simulink model "nonlinearstm_c"  (R2018b)
settings: configuration reference "Physics" (kept outside this file)
model workspace (MAT data in the model file):
  x0_positionstates = Simulink.Parameter
  x0_positionstates.Value = [0 0 0]
  x0_positionstates.DataType = 'auto'
  x0_positionstates.Dimensions = [1 3]
undefined symbols (not defined in the file): INIT__initialvalues__omega0_Wheels_radps__1, INIT__initialvalues__omega0_Wheels_radps__2, INIT__initialvalues__omega0_Wheels_radps__3, INIT__initialvalues__omega0_Wheels_radps__4, INIT__initialvalues__Vehicle_InitialVelocity_mps__1, INIT__initialvalues__Vehicle_InitialVelocity_mps__2, INIT__initialvalues__Vehicle_InitialYawRate_radps, x0_stm_vehiclestates
settings Model: DataDictionary=vehicleparameters_vehdynsim.sldd  OrderedModelArguments=off  Creator=wischnewski  LastModifiedBy=jens

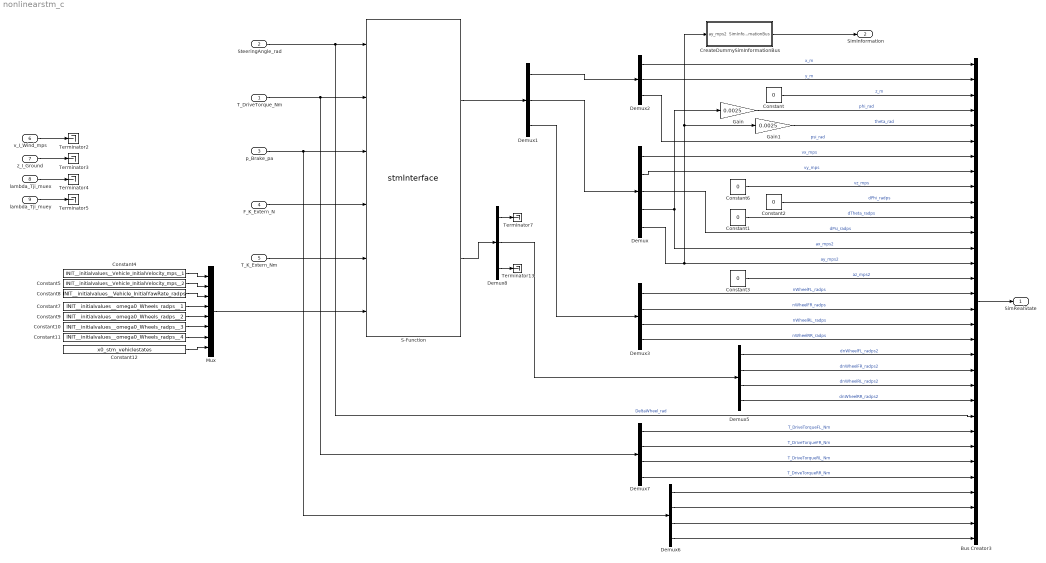
== system nonlinearstm_c ==
  T_DriveTorque_Nm : Inport
  SteeringAngle_rad : Inport  Port=2
  p_Brake_pa : Inport  Port=3
  F_K_Extern_N : Inport  Port=4  PortDimensions=3
  T_K_Extern_Nm : Inport  Port=5  PortDimensions=3
  v_I_Wind_mps : Inport  Port=6  PortDimensions=3
  z_I_Ground : Inport  Port=7  PortDimensions=4
  lambda_Tji_muex : Inport  Port=8  PortDimensions=4
  lambda_Tji_muey : Inport  Port=9  PortDimensions=4
  Bus Creator3 : BusCreator  Inputs=32  OutDataTypeStr=Bus: SimRealState
  Constant{,1..3,6} (5 alike) : Constant  Value=0
  Constant10 : Constant  Value=INIT__initialvalues__omega0_Wheels_radps__3
  Constant11 : Constant  Value=INIT__initialvalues__omega0_Wheels_radps__4
  Constant12 : Constant  Value=x0_stm_vehiclestates
  Constant4 : Constant  Value=INIT__initialvalues__Vehicle_InitialVelocity_mps__1
  Constant5 : Constant  Value=INIT__initialvalues__Vehicle_InitialVelocity_mps__2
  Constant7 : Constant  Value=INIT__initialvalues__omega0_Wheels_radps__1
  Constant8 : Constant  Value=INIT__initialvalues__Vehicle_InitialYawRate_radps
  Constant9 : Constant  Value=INIT__initialvalues__omega0_Wheels_radps__2
  CreateDummySimInformationBus : Subsystem
  Demux : Demux  Outputs=[1 1 1 1 1]
  Demux1 : Demux  Outputs=[3 5 4]
  Demux2 : Demux  Outputs=3
  Demux{3,5..7} (4 alike) : Demux
  Demux8 : Demux  Outputs=[6 4 8]
  Gain : Gain  Gain=0.0025
  Gain1 : Gain  Gain=0.0025
  Mux : Mux  Inputs=8
  S-Function : S-Function  FunctionName=stmInterface  SFunctionDeploymentMode=off  EnableBusSupport=off
  Terminator{2..5,7,13} (6 alike) : Terminator
  SimRealState : Outport  OutDataTypeStr=Bus: SimRealState
  SimInformation : Outport  Port=2  OutDataTypeStr=Bus: SimInformation
  wires:
  Demux/1 -> Bus Creator3/7  "vx_mps"
  Demux/2 -> Bus Creator3/8  "vy_mps"
  Demux2/3 -> Bus Creator3/6  "psi_rad"
  Demux/3 -> Bus Creator3/12  "dPsi_radps"
  Demux/4 -> Gain/1, Bus Creator3/13  "ax_mps2"
  Demux/5 -> Bus Creator3/14, CreateDummySimInformationBus/1(ay_mps2), Gain1/1  "ay_mps2"
  Demux2/1 -> Bus Creator3/1  "x_m"
  Demux2/2 -> Bus Creator3/2  "y_m"
  SteeringAngle_rad/1 -> Bus Creator3/24, S-Function/1  "DeltaWheel_rad"
  Bus Creator3/1 -> SimRealState/1
  Demux3/1 -> Bus Creator3/16  "nWheelFL_radps"
  Demux3/2 -> Bus Creator3/17  "nWheelFR_radps"
  Demux3/4 -> Bus Creator3/19  "nWheelRR_radps"
  Demux3/3 -> Bus Creator3/18  "nWheelRL_radps"
  Constant1/1 -> Bus Creator3/11  "dTheta_radps"
  Constant2/1 -> Bus Creator3/10  "dPhi_radps"
  Constant3/1 -> Bus Creator3/15  "az_mps2"
  Constant/1 -> Bus Creator3/3  "z_m"
  Gain1/1 -> Bus Creator3/5  "theta_rad"
  Gain/1 -> Bus Creator3/4  "phi_rad"
  Constant6/1 -> Bus Creator3/9  "vz_mps"
  T_DriveTorque_Nm/1 -> Demux7/1, S-Function/2
  p_Brake_pa/1 -> Demux6/1, S-Function/3
  v_I_Wind_mps/1 -> Terminator2/1
  z_I_Ground/1 -> Terminator3/1
  lambda_Tji_muex/1 -> Terminator4/1
  lambda_Tji_muey/1 -> Terminator5/1
  Demux5/2 -> Bus Creator3/21  "dnWheelFR_radps2"
  Demux5/3 -> Bus Creator3/22  "dnWheelRL_radps2"
  Demux5/4 -> Bus Creator3/23  "dnWheelRR_radps2"
  Demux5/1 -> Bus Creator3/20  "dnWheelFL_radps2"
  CreateDummySimInformationBus/1(SimInformationBus) -> SimInformation/1
  Demux7/1 -> Bus Creator3/25  "T_DriveTorqueFL_Nm"
  Demux7/2 -> Bus Creator3/26  "T_DriveTorqueFR_Nm"
  Demux7/3 -> Bus Creator3/27  "T_DriveTorqueRL_Nm"
  Demux7/4 -> Bus Creator3/28  "T_DriveTorqueRR_Nm"
  Demux6/1 -> Bus Creator3/29
  Demux6/2 -> Bus Creator3/30
  Demux6/3 -> Bus Creator3/31
  Demux6/4 -> Bus Creator3/32
  Mux/1 -> S-Function/6
  Constant5/1 -> Mux/2
  Constant4/1 -> Mux/1
  Constant8/1 -> Mux/3
  Constant7/1 -> Mux/4
  Constant9/1 -> Mux/5
  Constant10/1 -> Mux/6
  Constant11/1 -> Mux/7
  Constant12/1 -> Mux/8
  F_K_Extern_N/1 -> S-Function/4
  T_K_Extern_Nm/1 -> S-Function/5
  S-Function/1 -> Demux1/1
  Demux1/1 -> Demux2/1
  Demux1/2 -> Demux/1
  Demux1/3 -> Demux3/1
  S-Function/2 -> Demux8/1
  Demux8/1 -> Terminator7/1
  Demux8/3 -> Terminator13/1
  Demux8/2 -> Demux5/1

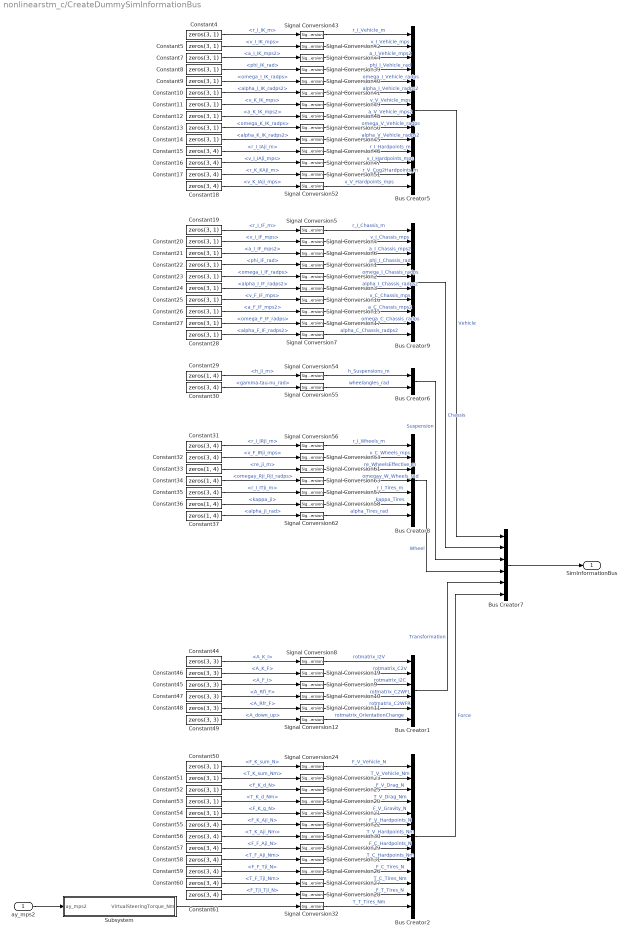
== system nonlinearstm_c/CreateDummySimInformationBus ==
  ay_mps2 : Inport
  Bus Creator1 : BusCreator  Inputs=6  OutDataTypeStr=Bus: Transformation
      settings: InheritFromInputs=off
  Bus Creator2 : BusCreator  Inputs=13  OutDataTypeStr=Bus: Force
      settings: InheritFromInputs=off
  Bus Creator5 : BusCreator  Inputs=14  OutDataTypeStr=Bus: Vehicle
      settings: InheritFromInputs=off
  Bus Creator6 : BusCreator  Inputs=2  OutDataTypeStr=Bus: Suspension
      settings: InheritFromInputs=off
  Bus Creator7 : BusCreator  Inputs=6  OutDataTypeStr=Bus: SimInformation
      settings: InheritFromInputs=off
  Bus Creator8 : BusCreator  Inputs=7  OutDataTypeStr=Bus: Wheel
      settings: InheritFromInputs=off
  Bus Creator9 : BusCreator  Inputs=10  OutDataTypeStr=Bus: Chassis
      settings: InheritFromInputs=off
  Constant{4..5,7..14,19..28,50..54} (25 alike) : Constant  Value=zeros(3, 1)
  Constant{15..18,30..32,35,55..61} (15 alike) : Constant  Value=zeros(3, 4)
  Constant{29,33..34,36..37} (5 alike) : Constant  Value=zeros(1, 4)
  Constant{44..49} (6 alike) : Constant  Value=zeros(3, 3)
  Signal Conversion{1..12,15..17,19..32,39..58,61..63} (52 alike) : SignalConversion  OverrideOpt=off
  Subsystem : Subsystem
  SimInformationBus : Outport
  wires:
  Signal Conversion46/1 -> Bus Creator5/11  "r_I_Hardpoints_m"
  Signal Conversion26/1 -> Bus Creator2/10  "F_C_Tires_N"
  Signal Conversion45/1 -> Bus Creator5/10  "alpha_V_Vehicle_radps2"
  Constant33/1 -> Signal Conversion61/1  "<re_ji_m>"
  Signal Conversion15/1 -> Bus Creator9/8  "a_C_Chassis_mps2"
  Signal Conversion58/1 -> Bus Creator8/6  "kappa_Tires"
  Constant60/1 -> Signal Conversion27/1  "<T_F_Tji_Nm>"
  Signal Conversion5/1 -> Bus Creator9/1  "r_I_Chassis_m"
  Signal Conversion17/1 -> Bus Creator9/9  "omega_C_Chassis_radps"
  Signal Conversion8/1 -> Bus Creator1/1  "rotmatrix_I2V"
  Constant13/1 -> Signal Conversion50/1  "<omega_K_IK_radps>"
  Constant24/1 -> Signal Conversion3/1  "<alpha_I_IF_radps2>"
  Signal Conversion16/1 -> Bus Creator9/7  "v_C_Chassis_mps"
  Signal Conversion23/1 -> Bus Creator2/2  "T_V_Vehicle_Nm"
  Signal Conversion3/1 -> Bus Creator9/6  "alpha_I_Chassis_radps2"
  Bus Creator5/1 -> Bus Creator7/1  "Vehicle"
  Signal Conversion32/1 -> Bus Creator2/13  "T_T_Tires_Nm"
  Signal Conversion39/1 -> Bus Creator5/4  "phi_I_Vehicle_rad"
  Signal Conversion29/1 -> Bus Creator2/8  "F_C_Hardpoints_N"
  Constant25/1 -> Signal Conversion16/1  "<v_F_IF_mps>"
  Signal Conversion43/1 -> Bus Creator5/1  "r_I_Vehicle_m"
  Constant47/1 -> Signal Conversion10/1  "<A_Rfl_F>"
  Constant9/1 -> Signal Conversion40/1  "<omega_I_IK_radps>"
  Constant26/1 -> Signal Conversion15/1  "<a_F_IF_mps2>"
  Constant27/1 -> Signal Conversion17/1  "<omega_F_IF_radps>"
  Signal Conversion10/1 -> Bus Creator1/4  "rotmatrix_C2WFL"
  Signal Conversion19/1 -> Bus Creator1/2  "rotmatrix_C2V"
  Constant7/1 -> Signal Conversion44/1  "<a_I_IK_mps2>"
  Bus Creator8/1 -> Bus Creator7/4  "Wheel"
  Signal Conversion9/1 -> Bus Creator1/3  "rotmatrix_I2C"
  Signal Conversion31/1 -> Bus Creator2/9  "T_C_Hardpoints_Nm"
  Signal Conversion62/1 -> Bus Creator8/7  "alpha_Tires_rad"
  Signal Conversion30/1 -> Bus Creator2/7  "T_V_Hardpoints_Nm"
  Signal Conversion48/1 -> Bus Creator5/8  "a_V_Vehicle_mps2"
  Signal Conversion54/1 -> Bus Creator6/1  "h_Suspensions_m"
  Signal Conversion56/1 -> Bus Creator8/1  "r_I_Wheels_m"
  Signal Conversion7/1 -> Bus Creator9/10  "alpha_C_Chassis_radps2"
  Signal Conversion12/1 -> Bus Creator1/6  "rotmatrix_OrientationChange"
  Signal Conversion21/1 -> Bus Creator2/5  "F_V_Gravity_N"
  Signal Conversion53/1 -> Bus Creator8/2  "v_C_Wheels_mps"
  Signal Conversion22/1 -> Bus Creator2/6  "F_V_Hardpoints_N"
  Signal Conversion27/1 -> Bus Creator2/11  "T_C_Tires_Nm"
  Signal Conversion51/1 -> Bus Creator5/13  "r_V_Cog2Hardpoints_m"
  Constant28/1 -> Signal Conversion7/1  "<alpha_F_IF_radps2>"
  Signal Conversion55/1 -> Bus Creator6/2  "wheelangles_rad"
  Signal Conversion57/1 -> Bus Creator8/5  "r_I_Tires_m"
  Signal Conversion4/1 -> Bus Creator9/2  "v_I_Chassis_mps"
  Bus Creator2/1 -> Bus Creator7/6  "Force"
  Signal Conversion20/1 -> Bus Creator2/4  "T_V_Drag_Nm"
  Signal Conversion40/1 -> Bus Creator5/5  "omega_I_Vehicle_radps"
  Bus Creator1/1 -> Bus Creator7/5  "Transformation"
  Signal Conversion41/1 -> Bus Creator5/6  "alpha_I_Vehicle_radps2"
  Bus Creator9/1 -> Bus Creator7/2  "Chassis"
  Signal Conversion6/1 -> Bus Creator9/3  "a_I_Chassis_mps2"
  Bus Creator6/1 -> Bus Creator7/3  "Suspension"
  Signal Conversion61/1 -> Bus Creator8/3  "re_WheelsEffective_m"
  Signal Conversion44/1 -> Bus Creator5/3  "a_I_Vehicle_mps2"
  Signal Conversion42/1 -> Bus Creator5/2  "v_I_Vehicle_mps"
  Signal Conversion63/1 -> Bus Creator8/4  "omegay_W_Wheels_rad"
  Constant31/1 -> Signal Conversion56/1  "<r_I_IRji_m>"
  Signal Conversion49/1 -> Bus Creator5/7  "v_V_Vehicle_mps"
  Signal Conversion28/1 -> Bus Creator2/12  "F_T_Tires_N"
  Signal Conversion11/1 -> Bus Creator1/5  "rotmatrix_C2WFR"
  Signal Conversion50/1 -> Bus Creator5/9  "omega_V_Vehicle_radps"
  Signal Conversion24/1 -> Bus Creator2/1  "F_V_Vehicle_N"
  Constant19/1 -> Signal Conversion5/1  "<r_I_IF_m>"
  Constant22/1 -> Signal Conversion1/1  "<phi_IF_rad>"
  Constant11/1 -> Signal Conversion49/1  "<v_K_IK_mps>"
  Constant58/1 -> Signal Conversion31/1  "<T_F_Aji_Nm>"
  Constant20/1 -> Signal Conversion4/1  "<v_I_IF_mps>"
  Constant44/1 -> Signal Conversion8/1  "<A_K_I>"
  Constant36/1 -> Signal Conversion58/1  "<kappa_ji>"
  Constant32/1 -> Signal Conversion53/1  "<v_F_IRji_mps>"
  Constant8/1 -> Signal Conversion39/1  "<phi_IK_rad>"
  Signal Conversion2/1 -> Bus Creator9/5  "omega_I_Chassis_radps"
  Constant5/1 -> Signal Conversion42/1  "<v_I_IK_mps>"
  Constant10/1 -> Signal Conversion41/1  "<alpha_I_IK_radps2>"
  Constant4/1 -> Signal Conversion43/1  "<r_I_IK_m>"
  Constant29/1 -> Signal Conversion54/1  "<h_ji_m>"
  Subsystem/1(VirtualSteeringTorque_Nm) -> Signal Conversion32/1
  Constant35/1 -> Signal Conversion57/1  "<r_I_ITji_m>"
  Signal Conversion47/1 -> Bus Creator5/12  "v_I_Hardpoints_mps"
  Constant57/1 -> Signal Conversion29/1  "<F_F_Aji_N>"
  Constant48/1 -> Signal Conversion11/1  "<A_Rfr_F>"
  Constant50/1 -> Signal Conversion24/1  "<F_K_sum_N>"
  Constant53/1 -> Signal Conversion20/1  "<T_K_d_Nm>"
  Constant49/1 -> Signal Conversion12/1  "<A_down_up>"
  Constant51/1 -> Signal Conversion23/1  "<T_K_sum_Nm>"
  Constant12/1 -> Signal Conversion48/1  "<a_K_IK_mps2>"
  Constant15/1 -> Signal Conversion46/1  "<r_I_IAji_m>"
  Constant54/1 -> Signal Conversion21/1  "<F_K_g_N>"
  Constant17/1 -> Signal Conversion51/1  "<r_K_KAji_m>"
  Constant55/1 -> Signal Conversion22/1  "<F_K_Aji_N>"
  Constant21/1 -> Signal Conversion6/1  "<a_I_IF_mps2>"
  Constant52/1 -> Signal Conversion25/1  "<F_K_d_N>"
  Constant30/1 -> Signal Conversion55/1  "<gamma-tau-nu_rad>"
  Constant14/1 -> Signal Conversion45/1  "<alpha_K_IK_radps2>"
  Constant18/1 -> Signal Conversion52/1  "<v_K_IAji_mps>"
  Constant59/1 -> Signal Conversion26/1  "<F_F_Tji_N>"
  Constant61/1 -> Signal Conversion28/1  "<F_Tji_Tji_N>"
  Constant56/1 -> Signal Conversion30/1  "<T_K_Aji_Nm>"
  Constant37/1 -> Signal Conversion62/1  "<alpha_ji_rad>"
  Constant34/1 -> Signal Conversion63/1  "<omegay_Rji_Rji_radps>"
  Constant45/1 -> Signal Conversion9/1  "<A_F_I>"
  Signal Conversion1/1 -> Bus Creator9/4  "phi_I_Chassis_rad"
  Signal Conversion52/1 -> Bus Creator5/14  "v_V_Hardpoints_mps"
  Constant46/1 -> Signal Conversion19/1  "<A_K_F>"
  Constant23/1 -> Signal Conversion2/1  "<omega_I_IF_radps>"
  Constant16/1 -> Signal Conversion47/1  "<v_I_IAji_mps>"
  Signal Conversion25/1 -> Bus Creator2/3  "F_V_Drag_N"
  Bus Creator7/1 -> SimInformationBus/1
  ay_mps2/1 -> Subsystem/1(ay_mps2)

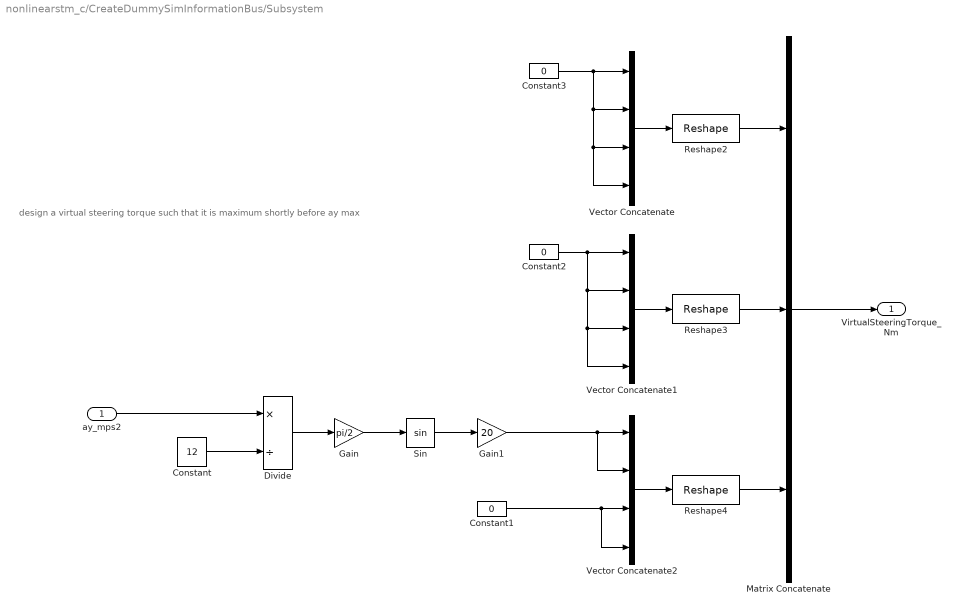
== system nonlinearstm_c/CreateDummySimInformationBus/Subsystem ==
  note: design a virtual steering torque such that it is maximum shortly before ay max
  ay_mps2 : Inport
  Constant : Constant  Value=12
  Constant1 : Constant  Value=0
  Constant2 : Constant  Value=0
  Constant3 : Constant  Value=0
  Divide : Product  Inputs=*/
  Gain : Gain  Gain=pi/2
  Gain1 : Gain  Gain=20
  Matrix Concatenate : Concatenate  NumInputs=3  Mode=Multidimensional array
  Reshape2 : Reshape  OutputDimensionality=Row vector (2-D)
  Reshape3 : Reshape  OutputDimensionality=Row vector (2-D)
  Reshape4 : Reshape  OutputDimensionality=Row vector (2-D)
  Sin : Trigonometry
  Vector Concatenate : Concatenate  NumInputs=4
  Vector Concatenate1 : Concatenate  NumInputs=4
  Vector Concatenate2 : Concatenate  NumInputs=4
  VirtualSteeringTorque_Nm : Outport
  wires:
  ay_mps2/1 -> Divide/1
  Constant/1 -> Divide/2
  Divide/1 -> Gain/1
  Gain/1 -> Sin/1
  Sin/1 -> Gain1/1
  Constant3/1 -> Vector Concatenate/4, Vector Concatenate/3, Vector Concatenate/2, Vector Concatenate/1
  Reshape3/1 -> Matrix Concatenate/2
  Reshape4/1 -> Matrix Concatenate/3
  Vector Concatenate1/1 -> Reshape3/1
  Constant1/1 -> Vector Concatenate2/4, Vector Concatenate2/3
  Vector Concatenate2/1 -> Reshape4/1
  Vector Concatenate/1 -> Reshape2/1
  Constant2/1 -> Vector Concatenate1/4, Vector Concatenate1/3, Vector Concatenate1/2, Vector Concatenate1/1
  Gain1/1 -> Vector Concatenate2/2, Vector Concatenate2/1
  Reshape2/1 -> Matrix Concatenate/1
  Matrix Concatenate/1 -> VirtualSteeringTorque_Nm/1
